simulink library "Coefficient_Evaluation_lib"  (Simulink 6.6)
libraries: aeroutilslib x1, simulink x1
settings Model: Creator=cbuttril  LastModifiedBy=cbuttril

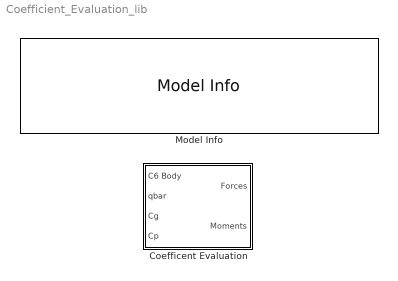
== system Coefficient_Evaluation_lib ==
  Coefficent Evaluation : Subsystem  mask{b=1, cbar=1, Sref=1}
      mask prompts: b "Reference Span (b)"; cbar "Reference Chord (cbar)"; Sref "Reference Area (Sref)"
      mask help:
      | Calulates the Force and Moments due to aerodynamic loads from vector of body axes aerodynamic coefficients:
      |    C6body = [Cx Cy Cz Cl Cm Cn].
      | Also requires dynamic pressure, cg/cp locations and reference lengths/area.
  Model Info : simulink/Model-Wide Utilities/Model Info  SystemSampleTime=-1  InitialBlockCM=None  BlockCM=None  Frame=on  DisplayStringWithTags=|  HorizontalTextAlignment=Center  LeftAlignmentValue=0.5  SourceBlockDiagram=Coefficient_Evaluation_lib  TagMaxNumber=20
      | Developed using Matlab Release 2007a
      | 
      | SVN:%<ModelVersion>
      | Last modifed by %<LastModifiedBy> on %<LastModificationDate>

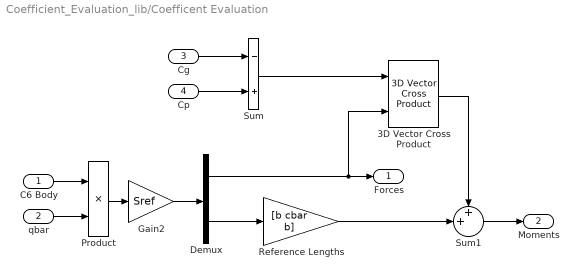
== system Coefficient_Evaluation_lib/Coefficent Evaluation ==
  C6 Body : Inport
  qbar : Inport  Port=2
  Cg : Inport  Port=3
  Cp : Inport  Port=4
  3D Vector Cross Product : aeroutilslib/3D Vector Cross Product  SystemSampleTime=-1
  Demux : Demux  Outputs=[3 3]
  Gain2 : Gain  Gain=Sref  SaturateOnIntegerOverflow=on
  Product : Product  SaturateOnIntegerOverflow=on  InputSameDT=on
  Reference Lengths : Gain  Gain=[b cbar b]  SaturateOnIntegerOverflow=on
  Sum : Sum  Inputs=-+  SaturateOnIntegerOverflow=on
  Sum1 : Sum  Inputs=++|  SaturateOnIntegerOverflow=on
  Forces : Outport
  Moments : Outport  Port=2
  wires:
  Sum/1 -> 3D Vector Cross Product/1
  Cg/1 -> Sum/1
  Cp/1 -> Sum/2
  C6 Body/1 -> Product/1
  qbar/1 -> Product/2
  Product/1 -> Gain2/1
  Gain2/1 -> Demux/1
  Demux/2 -> Reference Lengths/1
  Demux/1 -> 3D Vector Cross Product/2, Forces/1
  Reference Lengths/1 -> Sum1/2
  Sum1/1 -> Moments/1
  3D Vector Cross Product/1 -> Sum1/1
